simulink model "Etape3_bizarre"  (R2022a)
settings: Solver=VariableStepAuto  StartTime=0.0  StopTime=10.0  RelTol=1e-3
settings Model: Creator=mra4306  LastModifiedBy=mra4306

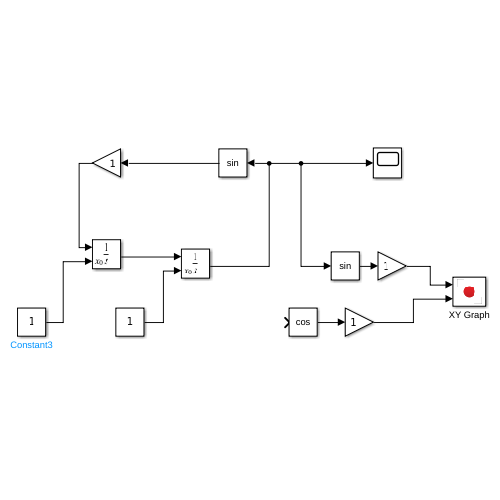
[thumbnail: Simulink's stored preview of the top-level diagram]
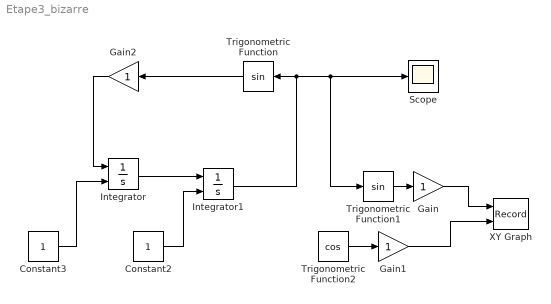
== system Etape3_bizarre ==
  Constant2 : Constant
  Constant3 : Constant
  Gain : Gain
  Gain1 : Gain
  Gain2 : Gain
  Integrator : Integrator  InitialConditionSource=external
  Integrator1 : Integrator  InitialConditionSource=external
  Scope : Scope
  Trigonometric Function : Trigonometry
  Trigonometric Function1 : Trigonometry
  Trigonometric Function2 : Trigonometry  Operator=cos
  XY Graph : Record  FileSettingsInternal="{\"entries\":[{\"content\":{\"excelSettings\":{\"content\":{},\"type\":\"Streamout.ExcelSettings\"}},\"type\":\"Streamout.FileSettingStorage\",\"uuid\":\"c281c875-2455-46b4-b612-08c43c0b9a6f\"}],\"packageUris\":[\"http://schema.mathworks.com/mf0/streamout_blocks/R2020a\"],\"version\":\"1.0\"}"  Layout=[1 1]  SignalsInternal="{\"entries\":[{\"content\":{\"signals\":[{\"content\":{\"blockPath\":[\"untitled1/XY Graph\"],\"channel\":[],\"dimensions\":[1],\"domain\":\"untitled1/XY Graph\",\"lineColor\":\"#a2142f\",\"plots\":[1],\"port\":1,\"sid\":[],\"signalID\":54,\"signalName\":\"XY Graph:1\"},\"type\":\"RecordBlkView.Signal\",\"uuid\":\"9b37b040-ec27-4abe-ae00-4ad27a288828\"},{\"content\":{\"blockPath\":[\"untitled1/XY Graph\"],\"channel\":[],\"dimensions\":[1],\"domain\":\"untitled1/XY Graph\",\"lineColor\":\"#139fff\",\"plots\":[1],\"port\":2,\"sid\":[],\"signalID\":57,\"signalName\":\"XY Graph:2\"},\"type\":\"RecordBlkView.Signal\",\"uuid\":\"684a05a5-cf06-4f66-93b6-23e6294ffdc5\"}]},\"type\":\"RecordBlkView.InputSignals\",\"uuid\":\"2619bf08-ba28-425a-9f81-a8e79f9c7cf5\"}],\"packageUris\":[\"http://schema.mathworks.com/mf0/streamout_blocks/R2020a\"],\"version\":\"1.0\"}"  VisualizationBindings="{\"xyplotplugin\":{\"info\":[{\"series\":[{\"bindingParametersList\":[{\"parameter\":\"X-Axis\",\"signalID\":54,\"signalName\":\"XY Graph:1\"},{\"parameter\":\"Y-Axis\",\"signalID\":57,\"signalName\":\"XY Graph:2\"}],\"seriesID\":44716}],\"subplotID\":1}]}}"  CompatibilityTag=XY
  wires:
  Trigonometric Function/1 -> Gain2/1
  Gain2/1 -> Integrator/1
  Constant3/1 -> Integrator/2
  Integrator/1 -> Integrator1/1
  Constant2/1 -> Integrator1/2
  Trigonometric Function1/1 -> Gain/1
  Trigonometric Function2/1 -> Gain1/1
  Gain/1 -> XY Graph/1
  Gain1/1 -> XY Graph/2
  Integrator1/1 -> Trigonometric Function1/1, Scope/1, Trigonometric Function/1
